simulink model "CommsOutCustom"  (R2026a)
settings: Solver=VariableStepAuto
libraries: etargetslib x1
settings Model: DataDictionary=QuadData.sldd  Creator=The MathWorks, Inc.  LastModifiedBy=The MathWorks, Inc.

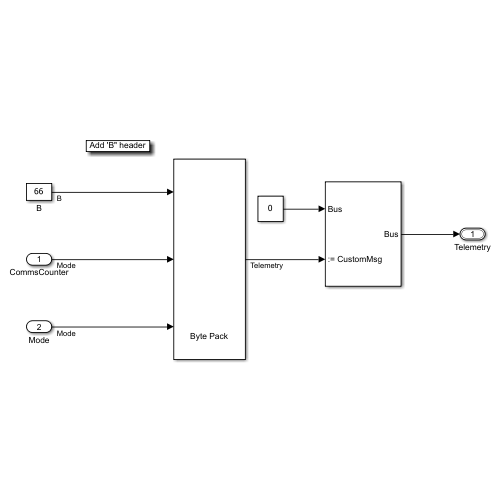
[thumbnail: Simulink's stored preview of the top-level diagram]
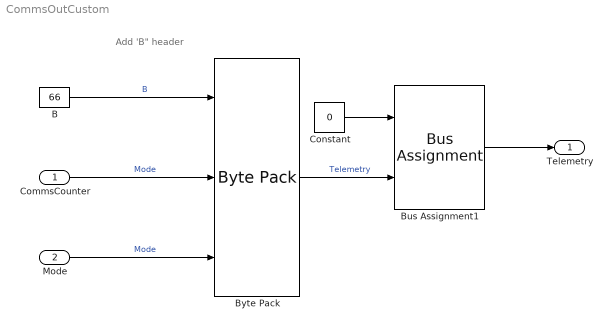
== system CommsOutCustom ==
  note: Add 'B" header
  CommsCounter : Inport  OutDataTypeStr=uint8  PortDimensions=1
  Mode : Inport  Port=2  OutDataTypeStr=uint8  PortDimensions=1
  B : Constant  Value=66  OutDataTypeStr=uint8  SampleTime=-1
  Bus Assignment1 : BusAssignment  AssignedSignals=CustomMsg
  Byte Pack : etargetslib/Byte Pack  datatypes={'uint8' 'uint8' 'uint8'}  byteAlign=1
  Constant : Constant  Value=0  OutDataTypeStr=Bus: Telemetry
  Telemetry : Outport  OutDataTypeStr=Bus: Telemetry
  wires:
  Mode/1 -> Byte Pack/3  "Mode"
  CommsCounter/1 -> Byte Pack/2  "Mode"
  B/1 -> Byte Pack/1  "B"
  Constant/1 -> Bus Assignment1/1
  Bus Assignment1/1 -> Telemetry/1
  Byte Pack/1 -> Bus Assignment1/2  "Telemetry"
